simulink model "ep3_2"  (R2018a)
settings: Solver=VariableStepAuto  StartTime=0.0  StopTime=10.0  RelTol=1e-3
libraries: simulink x1
settings Model: Creator=zheny  LastModifiedBy=zheny

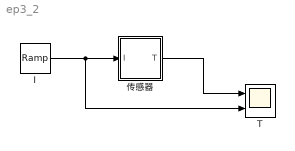
== system ep3_2 ==
  I : simulink/Sources/Ramp  slope=1  start=0  InitialOutput=0
  T : Scope  NumInputPorts=2
  传感器 : Subsystem  mask(ep3_2){Imin=-20, Imax=2, Tmin=-60, Tmax=100}
      mask help:
      | 该模型表示
      | T = (I-Imin)/(Imax-Imin).*(Tmax-Tmin)+Tmin;
      mask init:
      | I = 4:0.1:20;
      | Tmax = 40;
      | Tmin = 30;
      | Imax = 15;
      | Imin = 5;
      | T = (I-Imin)/(Imax-Imin).*(Tmax-Tmin)+Tmin;
      mask Help:
      | ep3_2
      | 该模型表示
      | T = (I-Imin)/(Imax-Imin).*(Tmax-Tmin)+Tmin;
      mask Display:
      | plot([0:0.1:1],[0:0.1:1])
      | port_label('input', 1, 'I')
      | port_label('output', 1, 'T')
  wires:
  I/1 -> T/2, 传感器/1(I)
  传感器/1(T) -> T/1

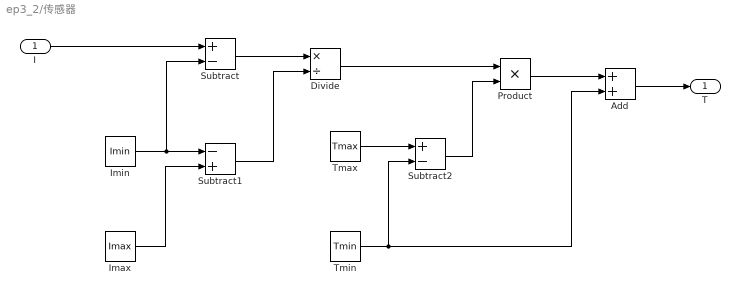
== system ep3_2/传感器 ==
  I : Inport
  Add : Sum
  Divide : Product  Inputs=*/
  Imax : Constant  Value=Imax
  Imin : Constant  Value=Imin
  Product : Product
  Subtract : Sum  Inputs=+-
  Subtract1 : Sum  Inputs=-+
  Subtract2 : Sum  Inputs=+-
  Tmax : Constant  Value=Tmax
  Tmin : Constant  Value=Tmin
  T : Outport
  wires:
  Subtract1/1 -> Divide/2
  Product/1 -> Add/1
  Imax/1 -> Subtract1/2
  Imin/1 -> Subtract/2, Subtract1/1
  Tmax/1 -> Subtract2/1
  Subtract/1 -> Divide/1
  Divide/1 -> Product/1
  Tmin/1 -> Add/2, Subtract2/2
  Subtract2/1 -> Product/2
  I/1 -> Subtract/1
  Add/1 -> T/1
